simulink model "inverted_pendulum_linear"  (R2020a)
settings: Solver=VariableStepAuto  StartTime=0.0  StopTime=10.0  RelTol=1e-3
settings Model: Creator=sidsu  LastModifiedBy=sidsu

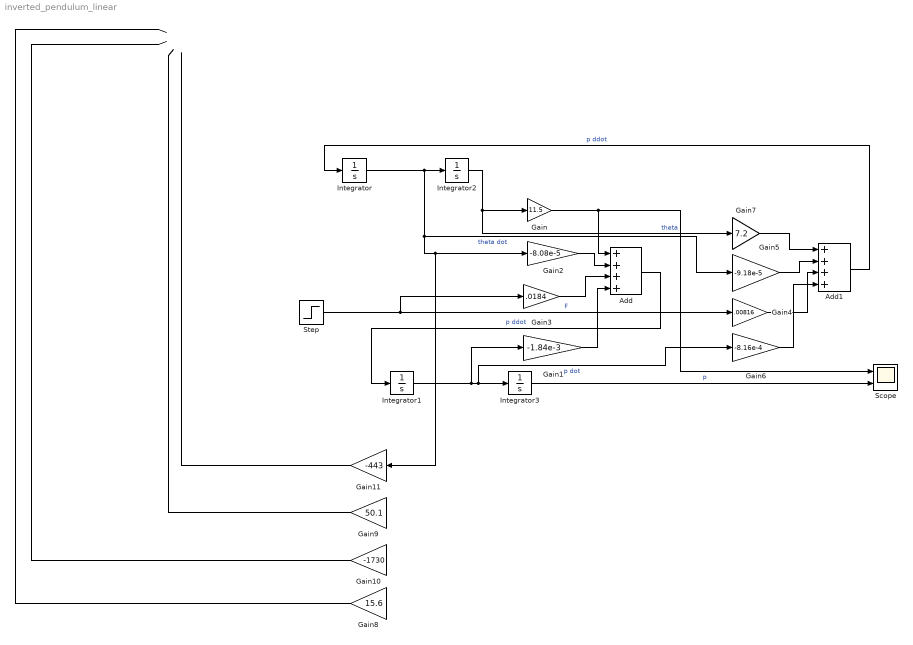
== system inverted_pendulum_linear ==
  Add : Sum  Inputs=++++
  Add1 : Sum  Inputs=++++
  Gain : Gain  Gain=11.5
  Gain1 : Gain  Gain=-1.84e-3
  Gain10 : Gain  Gain=-1730
  Gain11 : Gain  Gain=-443
  Gain2 : Gain  Gain=-8.08e-5
  Gain3 : Gain  Gain=.0184
  Gain4 : Gain  Gain=.00816
  Gain5 : Gain  Gain=-9.18e-5
  Gain6 : Gain  Gain=-8.16e-4
  Gain7 : Gain  Gain=7.2
  Gain8 : Gain  Gain=15.6
  Gain9 : Gain  Gain=50.1
  Integrator{,1..3} (4 alike) : Integrator
  Scope : Scope  NumInputPorts=2
  Step : Step  SampleTime=0
  wires:
  Integrator3/1 -> Scope/2  "p"
  Integrator1/1 -> Gain1/1, Gain6/1, Integrator3/1  "p dot"
  Integrator2/1 -> Gain7/1, Gain/1  "theta"
  Step/1 -> Gain3/1, Gain4/1  "F"
  Gain/1 -> Scope/1, Add/1
  Gain2/1 -> Add/2
  Gain3/1 -> Add/3
  Gain1/1 -> Add/4
  Add/1 -> Integrator1/1  "p ddot"
  Gain7/1 -> Add1/1
  Gain5/1 -> Add1/2
  Gain4/1 -> Add1/3
  Gain6/1 -> Add1/4
  Add1/1 -> Integrator/1  "p ddot"
  ? -> Gain8/1  "p"
  Gain11/1 -> ?
  Integrator/1 -> Gain11/1, Gain2/1, Gain5/1, Integrator2/1  "theta dot"
  Gain10/1 -> ?
  ? -> Gain10/1  "theta"
  Gain9/1 -> ?
  ? -> Gain9/1  "p ddot"
  Gain8/1 -> ?
